simulink model "test_Dynamics_coupled_full_temp"  (R2021b)
settings: Solver=VariableStepAuto  StartTime=0.0  StopTime=10.0  RelTol=1e-3
InitFcn:
  | % ************** Initiate forces
  | % f0=[0;0;0;0;0;0];
  | % f0=[0;0;0;0;0;0;0];
  | f_0=[0;0;0];
  | f_m=[0;0];
  | f_e=[0;0;0;0;0;0];
  | % ************** Initiate states
  | q_m=[0;0];
  | q_dot_m=[0;0];
  | P=[0;0;0];
  | V_I0=[0;0;0];
  | % ************** Load main
  | %run(Main.m)
values from neighbouring files (symbols this model uses):
  diag_M = diagonalize(M_frak0, M_frak)    [Create_Robot.m]    (also in Main.m; diagonalize.m = zeros(6*(n+1),6*(n+1)); test_C_Main.m)
  iota0 = [1 0 0; 0 1 0;zeros(3,3);0 0 1]    [Create_Robot.m]    (also in Main.m = eye(6,6); test_C_Main.m)
  Xi_m_matrix = zeros(6*n,n)    [Create_Robot.m]    (also in Main.m; test_C_Main.m)
undefined symbols (not defined in the file or in its folder): Xi_m
settings Model: Creator=Bmmog  LastModifiedBy=Bmmog
settings SolverCC: AllowMultiTaskInputOutput=on

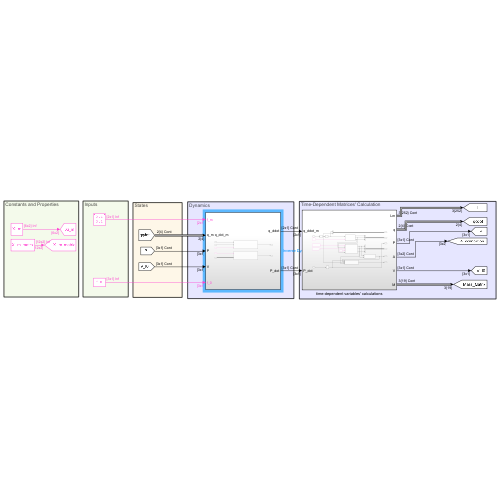
[thumbnail: Simulink's stored preview of the top-level diagram]
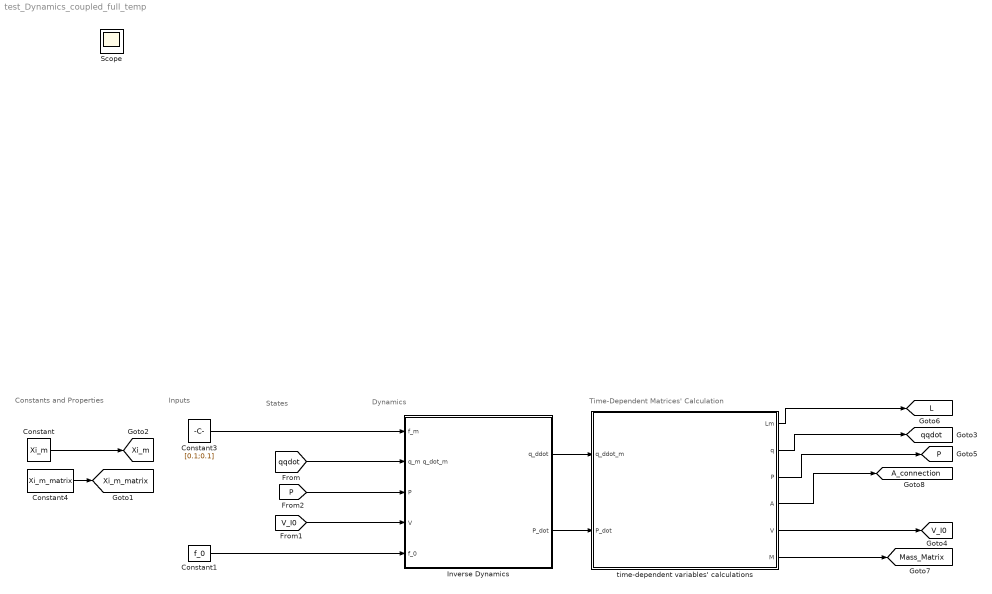
== system test_Dynamics_coupled_full_temp ==
  note: Time-Dependent Matrices' Calculation
  note: States
  note: Inputs
  note: Dynamics
  note: Constants and Properties
  Constant : Constant  Value=Xi_m  VectorParams1D=off
  Constant1 : Constant  Value=f_0  VectorParams1D=off
  Constant3 : Constant  Value=[0.1;0.1]  VectorParams1D=off
  Constant4 : Constant  Value=Xi_m_matrix  VectorParams1D=off
  Inverse Dynamics : Subsystem
  time-dependent variables' calculations : Subsystem
  Scope : Scope
  tag scope: A_connection=global, L=global, Mass_Matrix=global, P=global, V_I0=global, Xi_m=global, Xi_m_matrix=global, qqdot=global
  wires:
  Constant/1 -> [Xi_m]
  Constant4/1 -> [Xi_m_matrix]
  Constant3/1 -> Inverse Dynamics/1(f_m)
  time-dependent variables' calculations/6(M) -> [Mass_Matrix]
  time-dependent variables' calculations/1(Lm) -> [L]
  Inverse Dynamics/1(q_ddot) -> time-dependent variables' calculations/1(q_ddot_m)
  time-dependent variables' calculations/2(q) -> [qqdot]
  [qqdot] -> Inverse Dynamics/2(q_m q_dot_m)
  [V_I0] -> Inverse Dynamics/4(V)
  [P] -> Inverse Dynamics/3(P)
  time-dependent variables' calculations/3(P) -> [P]
  Constant1/1 -> Inverse Dynamics/5(f_0)
  time-dependent variables' calculations/4(A) -> [A_connection]
  time-dependent variables' calculations/5(V) -> [V_I0]
  Inverse Dynamics/2(P_dot) -> time-dependent variables' calculations/2(P_dot)

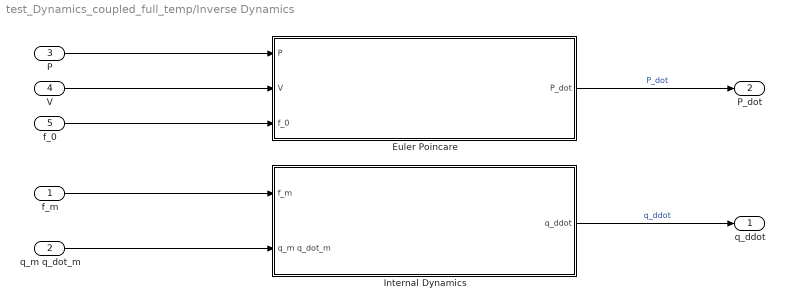
== system test_Dynamics_coupled_full_temp/Inverse Dynamics ==
  f_m : Inport
  q_m q_dot_m : Inport  Port=2
  P : Inport  Port=3
  V : Inport  Port=4
  f_0 : Inport  Port=5
  Euler Poincare : Subsystem
  Internal Dynamics : Subsystem
  q_ddot : Outport
  P_dot : Outport  Port=2
  wires:
  f_m/1 -> Internal Dynamics/1(f_m)
  Internal Dynamics/1(q_ddot) -> q_ddot/1  "q_ddot"
  q_m q_dot_m/1 -> Internal Dynamics/2(q_m q_dot_m)
  f_0/1 -> Euler Poincare/3(f_0)
  Euler Poincare/1(P_dot) -> P_dot/1  "P_dot"
  V/1 -> Euler Poincare/2(V)
  P/1 -> Euler Poincare/1(P)

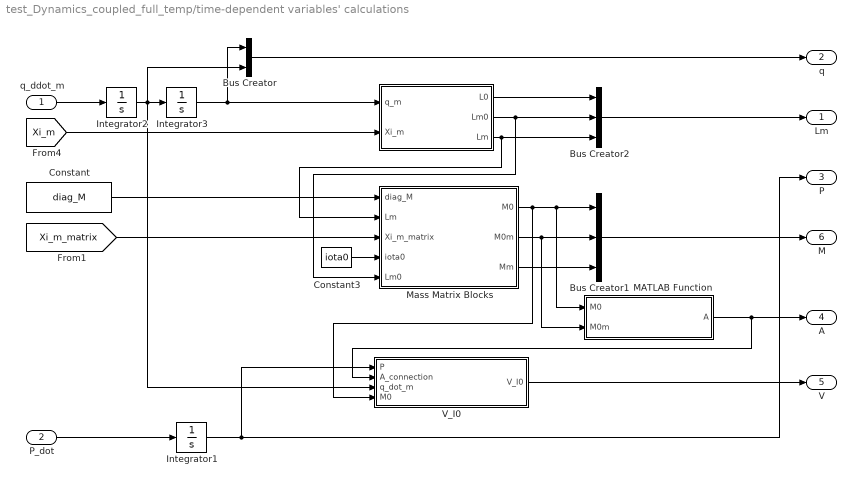
== system test_Dynamics_coupled_full_temp/time-dependent variables' calculations ==
  q_ddot_m : Inport
  P_dot : Inport  Port=2
  " " : MATLAB Function  TreatAsAtomicUnit=on
  Bus Creator : BusCreator  Inputs=2
  Bus Creator1 : BusCreator  Inputs=3
  Bus Creator2 : BusCreator  Inputs=3
  Constant : Constant  Value=diag_M  VectorParams1D=off
  Constant3 : Constant  Value=iota0  VectorParams1D=off
  Integrator1 : Integrator
  Integrator2 : Integrator
  Integrator3 : Integrator
  MATLAB Function : MATLAB Function  TreatAsAtomicUnit=on
  Mass Matrix Blocks : Subsystem
  V_I0 : MATLAB Function  TreatAsAtomicUnit=on
  Lm : Outport
  q : Outport  Port=2
  P : Outport  Port=3
  A : Outport  Port=4
  V : Outport  Port=5
  M : Outport  Port=6
  wires:
  Integrator2/1 -> V_I0/3(q_dot_m), Bus Creator/2, Integrator3/1
  q_ddot_m/1 -> Integrator2/1
  " "/1(L0) -> Bus Creator2/1
  " "/3(Lm) -> Mass Matrix Blocks/2(Lm), Bus Creator2/3
  " "/2(Lm0) -> Mass Matrix Blocks/5(Lm0), Bus Creator2/2
  Constant/1 -> Mass Matrix Blocks/1(diag_M)
  [Xi_m_matrix] -> Mass Matrix Blocks/3(Xi_m_matrix)
  [Xi_m] -> " "/2(Xi_m)
  Integrator3/1 -> Bus Creator/1, " "/1(q_m)
  Bus Creator/1 -> q/1
  Mass Matrix Blocks/1(M0) -> V_I0/4(M0), MATLAB Function/1(M0), Bus Creator1/1
  Mass Matrix Blocks/3(Mm) -> Bus Creator1/3
  Bus Creator1/1 -> M/1
  Mass Matrix Blocks/2(M0m) -> MATLAB Function/2(M0m), Bus Creator1/2
  MATLAB Function/1(A) -> V_I0/2(A_connection), A/1
  Constant3/1 -> Mass Matrix Blocks/4(iota0)
  Bus Creator2/1 -> Lm/1
  Integrator1/1 -> V_I0/1(P), P/1
  P_dot/1 -> Integrator1/1
  V_I0/1(V_I0) -> V/1

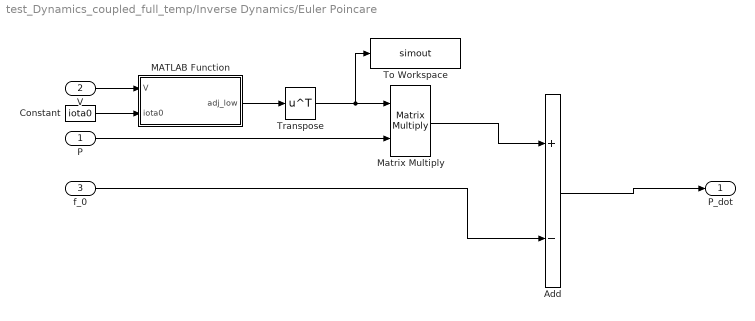
== system test_Dynamics_coupled_full_temp/Inverse Dynamics/Euler Poincare ==
  P : Inport
  V : Inport  Port=2
  f_0 : Inport  Port=3
  Add : Sum  Inputs=+-
  Constant : Constant  Value=iota0
  MATLAB Function : MATLAB Function  TreatAsAtomicUnit=on
  Matrix Multiply : Product  Multiplication=Matrix(*)
  To Workspace : ToWorkspace  VariableName=simout  SaveFormat=Timeseries  SampleTime=-1
  Transpose : Math  Operator=transpose  SaturateOnIntegerOverflow=on
  P_dot : Outport
  wires:
  P/1 -> Matrix Multiply/2
  MATLAB Function/1(adj_low) -> Transpose/1
  V/1 -> MATLAB Function/1(V)
  Transpose/1 -> To Workspace/1, Matrix Multiply/1
  Matrix Multiply/1 -> Add/1
  f_0/1 -> Add/2
  Add/1 -> P_dot/1
  Constant/1 -> MATLAB Function/2(iota0)

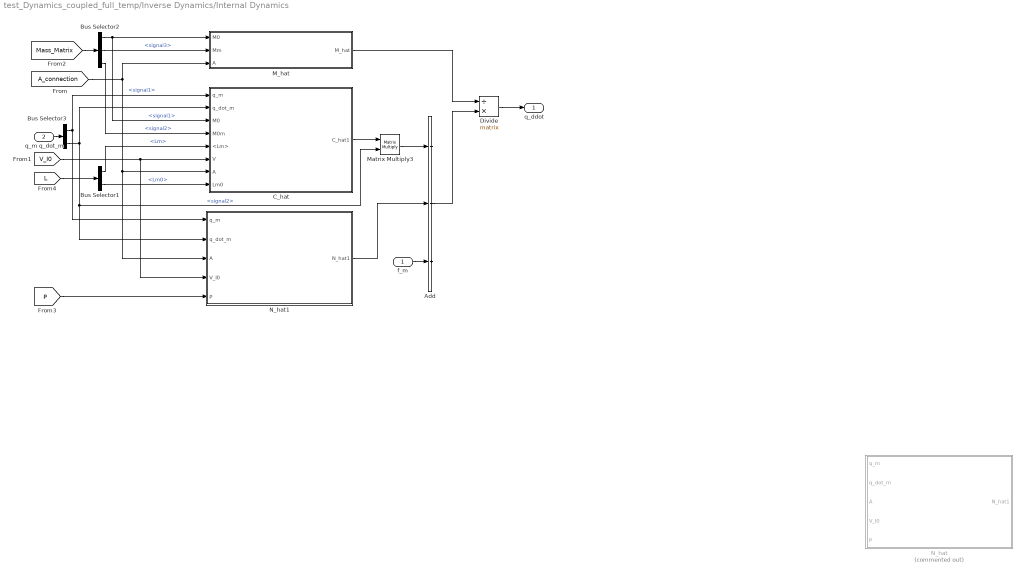
== system test_Dynamics_coupled_full_temp/Inverse Dynamics/Internal Dynamics ==
  f_m : Inport
  q_m q_dot_m : Inport  Port=2
  Add : Sum  Inputs=--+
  Bus Selector1 : BusSelector  OutputSignals=Lm,Lm0
  Bus Selector2 : BusSelector  OutputSignals=signal1,signal3,signal2
  Bus Selector3 : BusSelector  OutputSignals=signal1,signal2
  C_hat : Subsystem
  Divide : Product  Inputs=/*  Multiplication=Matrix(*)
  M_hat : MATLAB Function  TreatAsAtomicUnit=on
  Matrix Multiply3 : Product  Multiplication=Matrix(*)
  N_hat : Subsystem  Commented=on
  N_hat1 : Subsystem
  q_ddot : Outport
  wires:
  f_m/1 -> Add/3
  Divide/1 -> q_ddot/1
  q_m q_dot_m/1 -> Bus Selector3/1
  [Mass_Matrix] -> Bus Selector2/1
  [L] -> Bus Selector1/1
  C_hat/1(C_hat1) -> Matrix Multiply3/1
  Matrix Multiply3/1 -> Add/1
  Add/1 -> Divide/2
  Bus Selector3/2 -> C_hat/2(q_dot_m), N_hat1/2(q_dot_m), Matrix Multiply3/2  "<signal2>"
  Bus Selector3/1 -> C_hat/1(q_m), N_hat1/1(q_m)  "<signal1>"
  Bus Selector1/1 -> C_hat/5(<Lm>)  "<Lm>"
  M_hat/1(M_hat) -> Divide/1
  Bus Selector2/1 -> M_hat/1(M0), C_hat/3(M0)  "<signal1>"
  Bus Selector2/2 -> M_hat/2(Mm)  "<signal3>"
  [A_connection] -> N_hat1/3(A), C_hat/7(A), M_hat/3(A)
  Bus Selector2/3 -> C_hat/4(M0m)  "<signal2>"
  [V_I0] -> C_hat/6(V), N_hat1/4(V_I0)
  Bus Selector1/2 -> C_hat/8(Lm0)  "<Lm0>"
  [P] -> N_hat1/5(P)
  N_hat1/1(N_hat1) -> Add/2

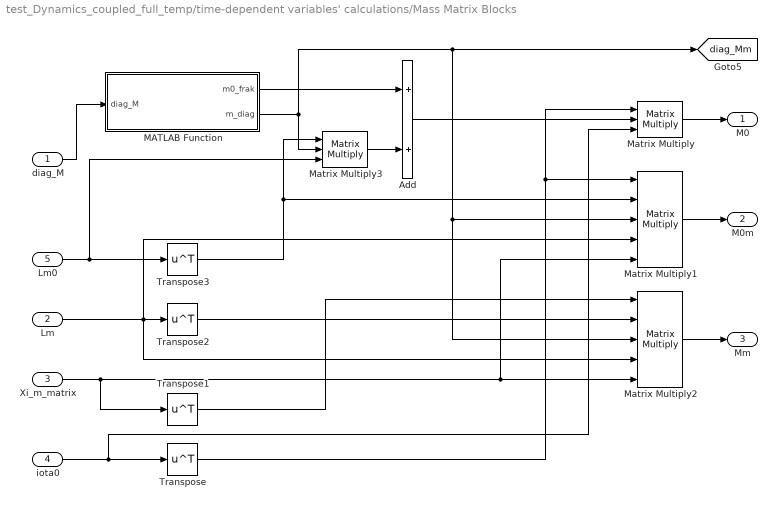
== system test_Dynamics_coupled_full_temp/time-dependent variables' calculations/Mass Matrix Blocks ==
  diag_M : Inport
  Lm : Inport  Port=2
  Xi_m_matrix : Inport  Port=3
  iota0 : Inport  Port=4
  Lm0 : Inport  Port=5
  Add : Sum
  MATLAB Function : MATLAB Function  TreatAsAtomicUnit=on
  Matrix Multiply : Product  Inputs=3  Multiplication=Matrix(*)
  Matrix Multiply1 : Product  Inputs=5  Multiplication=Matrix(*)
  Matrix Multiply2 : Product  Inputs=5  Multiplication=Matrix(*)
  Matrix Multiply3 : Product  Inputs=3  Multiplication=Matrix(*)
  Transpose{,1..3} (4 alike) : Math  Operator=transpose  SaturateOnIntegerOverflow=on
  M0 : Outport
  M0m : Outport  Port=2
  Mm : Outport  Port=3
  tag scope: diag_Mm=global
  wires:
  Matrix Multiply2/1 -> Mm/1
  Xi_m_matrix/1 -> Transpose1/1, Matrix Multiply1/5, Matrix Multiply2/5
  diag_M/1 -> MATLAB Function/1(diag_M)
  Lm/1 -> Matrix Multiply2/4, Matrix Multiply1/4, Transpose2/1
  Transpose1/1 -> Matrix Multiply2/1
  Transpose2/1 -> Matrix Multiply2/2
  MATLAB Function/2(m_diag) -> Matrix Multiply1/3, Matrix Multiply2/3, [diag_Mm], Matrix Multiply3/2
  Matrix Multiply1/1 -> M0m/1
  Matrix Multiply/1 -> M0/1
  iota0/1 -> Matrix Multiply/3, Transpose/1
  Transpose/1 -> Matrix Multiply/1, Matrix Multiply1/1
  Add/1 -> Matrix Multiply/2
  Matrix Multiply3/1 -> Add/2
  MATLAB Function/1(m0_frak) -> Add/1
  Lm0/1 -> Matrix Multiply3/3, Transpose3/1
  Transpose3/1 -> Matrix Multiply1/2, Matrix Multiply3/1

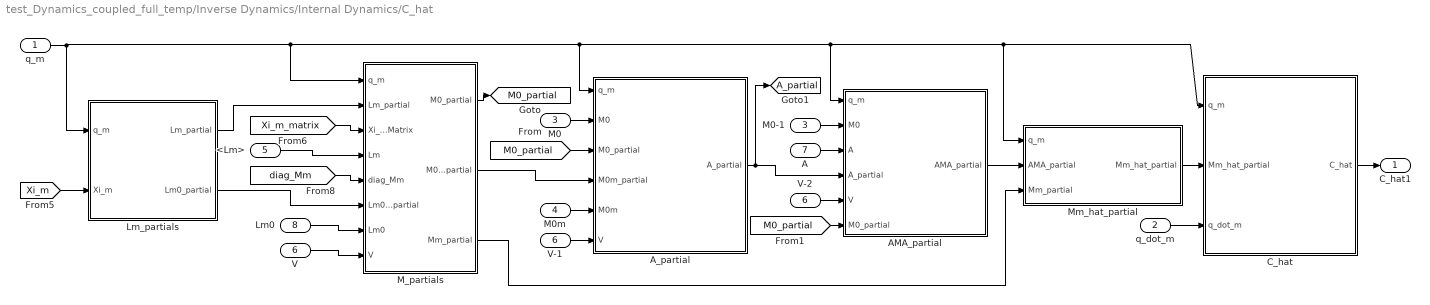
== system test_Dynamics_coupled_full_temp/Inverse Dynamics/Internal Dynamics/C_hat ==
  q_m : Inport
  q_dot_m : Inport  Port=2
  M0 : Inport  Port=3
  M0m : Inport  Port=4
  <Lm> : Inport  Port=5
  V : Inport  Port=6
  A : Inport  Port=7
  Lm0 : Inport  Port=8
  AMA_partial : MATLAB Function  TreatAsAtomicUnit=on
  A_partial : MATLAB Function  TreatAsAtomicUnit=on
  C_hat : MATLAB Function  TreatAsAtomicUnit=on
  Lm_partials : Subsystem
  M0-1 : InportShadow  Port=3
  M_partials : Subsystem
  Mm_hat_partial : MATLAB Function  TreatAsAtomicUnit=on
  V-1 : InportShadow  Port=6
  V-2 : InportShadow  Port=6
  C_hat1 : Outport
  tag scope: A_partial=global, M0_partial=global
  wires:
  C_hat/1(C_hat) -> C_hat1/1
  q_m/1 -> Mm_hat_partial/1(q_m), C_hat/1(q_m), AMA_partial/1(q_m), A_partial/1(q_m), M_partials/1(q_m), Lm_partials/1(q_m)
  q_dot_m/1 -> C_hat/3(q_dot_m)
  [Xi_m_matrix] -> M_partials/3(Xi_m_Matrix)
  <Lm>/1 -> M_partials/4(Lm)
  [diag_Mm] -> M_partials/5(diag_Mm)
  [Xi_m] -> Lm_partials/2(Xi_m)
  Lm_partials/1(Lm_partial) -> M_partials/2(Lm_partial)
  M_partials/3(Mm_partial) -> Mm_hat_partial/3(Mm_partial)
  Mm_hat_partial/1(Mm_hat_partial) -> C_hat/2(Mm_hat_partial)
  AMA_partial/1(AMA_partial) -> Mm_hat_partial/2(AMA_partial)
  A_partial/1(A_partial) -> [A_partial], AMA_partial/4(A_partial)
  M0/1 -> A_partial/2(M0)
  M0m/1 -> A_partial/5(M0m)
  V/1 -> M_partials/8(V)
  M_partials/2(M0m_partial) -> A_partial/4(M0m_partial)
  A/1 -> AMA_partial/3(A)
  Lm_partials/2(Lm0_partial) -> M_partials/6(Lm0_partial)
  Lm0/1 -> M_partials/7(Lm0)
  V-1/1 -> A_partial/6(V)
  V-2/1 -> AMA_partial/5(V)
  M0-1/1 -> AMA_partial/2(M0)
  M_partials/1(M0_partial) -> [M0_partial]
  [M0_partial] -> A_partial/3(M0_partial)
  [M0_partial] -> AMA_partial/6(M0_partial)

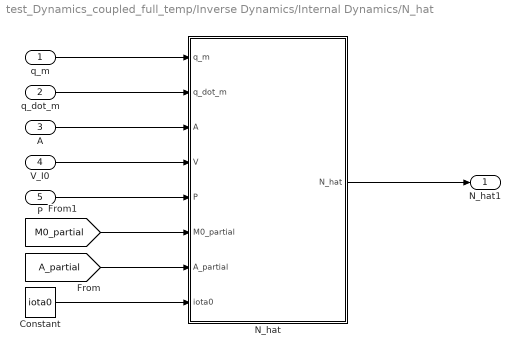
== system test_Dynamics_coupled_full_temp/Inverse Dynamics/Internal Dynamics/N_hat ==
  q_m : Inport
  q_dot_m : Inport  Port=2
  A : Inport  Port=3
  V_I0 : Inport  Port=4
  P : Inport  Port=5
  Constant : Constant  Value=iota0
  N_hat : MATLAB Function  TreatAsAtomicUnit=on
  N_hat1 : Outport
  wires:
  P/1 -> N_hat/5(P)
  [M0_partial] -> N_hat/6(M0_partial)
  N_hat/1(N_hat) -> N_hat1/1
  q_m/1 -> N_hat/1(q_m)
  q_dot_m/1 -> N_hat/2(q_dot_m)
  V_I0/1 -> N_hat/4(V)
  A/1 -> N_hat/3(A)
  [A_partial] -> N_hat/7(A_partial)
  Constant/1 -> N_hat/8(iota0)

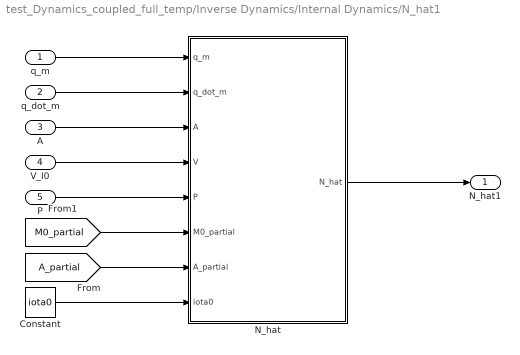
== system test_Dynamics_coupled_full_temp/Inverse Dynamics/Internal Dynamics/N_hat1 ==
  q_m : Inport
  q_dot_m : Inport  Port=2
  A : Inport  Port=3
  V_I0 : Inport  Port=4
  P : Inport  Port=5
  Constant : Constant  Value=iota0
  N_hat : MATLAB Function  TreatAsAtomicUnit=on
  N_hat1 : Outport
  wires:
  P/1 -> N_hat/5(P)
  [M0_partial] -> N_hat/6(M0_partial)
  N_hat/1(N_hat) -> N_hat1/1
  q_m/1 -> N_hat/1(q_m)
  q_dot_m/1 -> N_hat/2(q_dot_m)
  V_I0/1 -> N_hat/4(V)
  A/1 -> N_hat/3(A)
  [A_partial] -> N_hat/7(A_partial)
  Constant/1 -> N_hat/8(iota0)

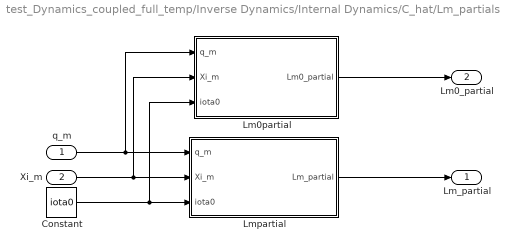
== system test_Dynamics_coupled_full_temp/Inverse Dynamics/Internal Dynamics/C_hat/Lm_partials ==
  q_m : Inport
  Xi_m : Inport  Port=2
  Constant : Constant  Value=iota0
  Lm0partial : MATLAB Function  TreatAsAtomicUnit=on
  Lmpartial : MATLAB Function  TreatAsAtomicUnit=on
  Lm_partial : Outport
  Lm0_partial : Outport  Port=2
  wires:
  Xi_m/1 -> Lm0partial/2(Xi_m), Lmpartial/2(Xi_m)
  q_m/1 -> Lm0partial/1(q_m), Lmpartial/1(q_m)
  Lmpartial/1(Lm_partial) -> Lm_partial/1
  Constant/1 -> Lm0partial/3(iota0), Lmpartial/3(iota0)
  Lm0partial/1(Lm0_partial) -> Lm0_partial/1

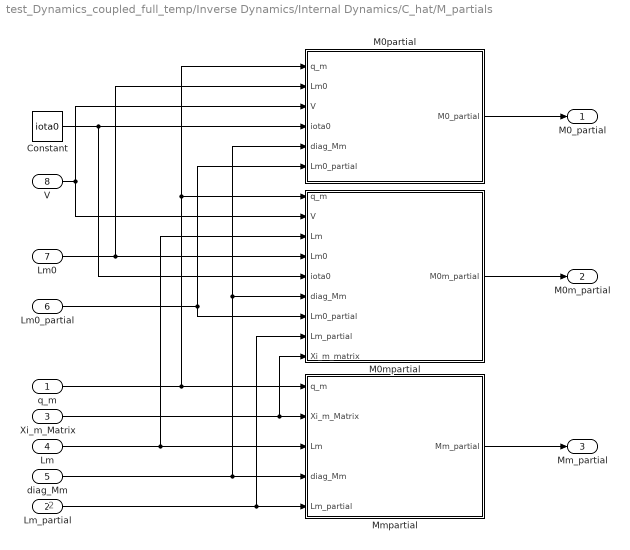
== system test_Dynamics_coupled_full_temp/Inverse Dynamics/Internal Dynamics/C_hat/M_partials ==
  note: 2
  q_m : Inport
  Lm_partial : Inport  Port=2
  Xi_m_Matrix : Inport  Port=3
  Lm : Inport  Port=4
  diag_Mm : Inport  Port=5
  Lm0_partial : Inport  Port=6
  Lm0 : Inport  Port=7
  V : Inport  Port=8
  " M0partial" : MATLAB Function  TreatAsAtomicUnit=on
  Constant : Constant  Value=iota0
  M0mpartial : MATLAB Function  TreatAsAtomicUnit=on
  Mmpartial : MATLAB Function  TreatAsAtomicUnit=on
  M0_partial : Outport
  M0m_partial : Outport  Port=2
  Mm_partial : Outport  Port=3
  wires:
  Xi_m_Matrix/1 -> M0mpartial/9(Xi_m_matrix), Mmpartial/2(Xi_m_Matrix)
  Lm/1 -> M0mpartial/3(Lm), Mmpartial/3(Lm)
  Mmpartial/1(Mm_partial) -> Mm_partial/1
  diag_Mm/1 -> " M0partial"/5(diag_Mm), M0mpartial/6(diag_Mm), Mmpartial/4(diag_Mm)
  M0mpartial/1(M0m_partial) -> M0m_partial/1
  Lm_partial/1 -> M0mpartial/8(Lm_partial), Mmpartial/5(Lm_partial)
  q_m/1 -> " M0partial"/1(q_m), M0mpartial/1(q_m), Mmpartial/1(q_m)
  " M0partial"/1(M0_partial) -> M0_partial/1
  Constant/1 -> " M0partial"/4(iota0), M0mpartial/5(iota0)
  Lm0_partial/1 -> " M0partial"/6(Lm0_partial), M0mpartial/7(Lm0_partial)
  Lm0/1 -> " M0partial"/2(Lm0), M0mpartial/4(Lm0)
  V/1 -> M0mpartial/2(V), " M0partial"/3(V)

== matlab function test_Dynamics_coupled_full_temp/time-dependent variables' calculations/MATLAB Function ==
  data: M0 input; M0m input; A output
function A=A_connection(M0,M0m)
% Compute the connection A from mass properties

A=M0\M0m;

== matlab function test_Dynamics_coupled_full_temp/Inverse Dynamics/Internal Dynamics/C_hat/Lm_partials/Lmpartial ==
  data: q_m input; Lm_partial output; Xi_m input; iota0 input
function Lm_partial  = Lm_partial(q_m,Xi_m,iota0)
% Calculates the C_hat_m matrix from base pose and arm joint angles

n=length(q_m);

% Find partial of Lm0 to joint angles
Lm_partial=zeros(6*n,6*n,n); % 6nx6xn
for i=1:n
    for j=1:n
        for k=1:n
            if j==k
                Lm_partial(6*(j-1)+1:6*(j-1)+6,6*(k-1)+1:6*(k-1)+6,i)=eye(6,6);
            elseif j>i && i>=k
                Lm_partial(6*(j-1)+1:6*j,6*(k-1)+1:6*k,i)=-Ad_frak(j,i+1,Xi_m,q_m)*adjoint_low(Xi_m(:,i),iota0)*Ad_frak(i,k,Xi_m,q_m); % equation 81 of TRO paper
            elseif i==j && i>=k
                Lm_partial(6*(j-1)+1:6*j,6*(k-1)+1:6*k,i)=-adjoint_low(Xi_m(:,i),iota0)*Ad_frak(i,k,Xi_m,q_m); % equation 81 of TRO paper
            else
                Lm_partial(6*(j-1)+1:6*(j-1)+6,6*(k-1)+1:6*(k-1)+6,i)=zeros(6,6);
            end

        end
    end
end

== matlab function test_Dynamics_coupled_full_temp/Inverse Dynamics/Internal Dynamics/C_hat/M_partials/ M0partial ==
  data: q_m input; M0_partial output; Lm0 input; V input; iota0 input; diag_Mm input; Lm0_partial input
function M0_partial = M0_partial(q_m,Lm0,V,iota0,diag_Mm,Lm0_partial)
% Calculates the C_hat_m matrix from base pose and arm joint angles

n=length(q_m);
b=length(V);

% Find partial of M0 to joint angles
M0_partial=zeros(b,b,n); %initiate
for i=1:n
    M0_partial(1:b,1:b,i)= iota0'*(transpose(Lm0_partial(1:end,1:end,i))*diag_Mm*Lm0+transpose(Lm0)*diag_Mm*Lm0_partial(1:end,1:end,i))*iota0; %6x6 %equation 117 of TRO
end

== matlab function test_Dynamics_coupled_full_temp/Inverse Dynamics/Internal Dynamics/C_hat/M_partials/M0mpartial ==
  data: q_m input; M0m_partial output; V input; Lm input; Lm0 input; iota0 input; diag_Mm input; Lm0_partial input; Lm_partial input; Xi_m_matrix input
function M0m_partial = M0m_partial(q_m,V,Lm,Lm0,iota0,diag_Mm,Lm0_partial,Lm_partial, Xi_m_matrix)
% Calculates the C_hat_m matrix from base pose and arm joint angles

n=length(q_m);
b=length(V);

% Find partial of M0m to joint angles
M0m_partial=zeros(b,n,n);
for i=1:n
    M0m_partial(1:b,1:n,i)= iota0'*((transpose(Lm0_partial(1:end,1:end,i))*diag_Mm*Lm+transpose(Lm0)*diag_Mm*Lm_partial(1:end,1:end,i)))*Xi_m_matrix; % equation 118 of TRO paper
end

== matlab function test_Dynamics_coupled_full_temp/time-dependent variables' calculations/Mass Matrix Blocks/MATLAB Function ==
  data: diag_M input; m0_frak output; m_diag output
function [m0_frak,m_diag]=m_frak_decomp(diag_M)
% Compute the Mass Matrix of the multibody system.
%   Output:
%   M0      Spacecraft mass matrix 
%   M0m
%   Mm      Manipulator mass matrix

%n=length(q_m);

m0_frak=diag_M(1:6,1:6);
m_diag=diag_M(7:end,7:end);

== matlab function test_Dynamics_coupled_full_temp/Inverse Dynamics/Internal Dynamics/C_hat/A_partial ==
  data: q_m input; A_partial output; M0 input; M0_partial input; M0m_partial input; M0m input; V input
function A_partial = A_partial(q_m,M0,M0_partial,M0m_partial,M0m,V)
% Calculates the C_hat_m matrix from base pose and arm joint angles

n=length(q_m);
b=length(V);

% Find partial of connection A to each joint angle
A_partial=zeros(b,n,n);

temp1=zeros(b,n);
temp2=zeros(b,n);
temp3=zeros(b,n);

for i=1:n
    temp1=M0\M0_partial(1:b,1:b,i);
    temp2=M0\M0m;
    temp3=M0\M0m_partial(1:b,1:n,i);
    A_partial(1:b,1:n,i)=temp1*temp2+temp3; % Equation 122
end

== matlab function test_Dynamics_coupled_full_temp/Inverse Dynamics/Internal Dynamics/C_hat/M_partials/Mmpartial ==
  data: q_m input; Mm_partial output; Xi_m_Matrix input; Lm input; diag_Mm input; Lm_partial input
function Mm_partial = Mm_partial(q_m,Xi_m_Matrix,Lm,diag_Mm,Lm_partial)
% Calculates the C_hat_m matrix from base pose and arm joint angles

n=length(q_m);

% find the non-generalized arm mass matrix'x derivative to joint angles
Mm_partial=zeros(n,n,n);
for i=1:n
    Mm_partial(1:n,1:n,i)=transpose(Xi_m_Matrix)*(transpose(Lm_partial(1:6*n,1:6*n,i))*diag_Mm*Lm + ...
        transpose(Lm)*diag_Mm*Lm_partial(1:6*n,1:6*n,i))*Xi_m_Matrix; %calcualte the derivative of not-augmented arm mass matrix from equation 120 of TRO paper
end

== matlab function test_Dynamics_coupled_full_temp/Inverse Dynamics/Internal Dynamics/C_hat/AMA_partial ==
  data: q_m input; AMA_partial output; M0 input; A input; A_partial input; V input; M0_partial input
function AMA_partial = AMA_partial(q_m,M0,A,A_partial,V,M0_partial)
% Calculates the C_hat_m matrix from base pose and arm joint angles

n=length(q_m);
b=length(V);

% find the temp intermediate term
AMA_partial=zeros(n,n,n);
for i=1:n
    AMA_partial(1:n,1:n,i)=transpose(A_partial(1:b,1:n,i))*M0*A+transpose(A)*M0_partial(1:b,1:b,i)*A+transpose(A)*M0*A_partial(1:b,1:n,i); %calcualte the derivative of not-augmented arm mass matrix from equation 121 of TRO paper
end

== matlab function test_Dynamics_coupled_full_temp/Inverse Dynamics/Internal Dynamics/C_hat/Mm_hat_partial ==
  data: q_m input; AMA_partial input; Mm_hat_partial output; Mm_partial input
function Mm_hat_partial = Mm_hat_partial(q_m, AMA_partial, Mm_partial)
% Calculates the C_hat_m matrix from base pose and arm joint angles

n=length(q_m);

% find the generalized arm mass matrix'x derivative to joint angles
Mm_hat_partial=zeros(n,n,n);
for i=1:n
    Mm_hat_partial(1:n,1:n,i)=Mm_partial(1:n,1:n,i)-AMA_partial(1:n,1:n,i); %calcualte the derivative of augmented arm mass matrix from equation 119 of TRO paper
end

== matlab function test_Dynamics_coupled_full_temp/time-dependent variables' calculations/V_I0 ==
  data: P input; A_connection input; q_dot_m input; M0 input; V_I0 output
function V_I0=V_I0(P,A_connection,q_dot_m,M0)
% Find the spaccecraft velocity V_I0
% M0_inv=inv(M0);
% temp=P-transpose(A_connection)*q_dot_m;
V_I0=M0\P-A_connection*q_dot_m;

== matlab function test_Dynamics_coupled_full_temp/Inverse Dynamics/Internal Dynamics/N_hat1/N_hat ==
  data: N_hat output; q_m input; q_dot_m input; A input; V input; P input; M0_partial input; A_partial input; iota0 input
function N_hat = N_hat(q_m,q_dot_m,A,V,P,M0_partial, A_partial, iota0)
% Calculates the N_hat_m matrix from base pose and arm joint angles

n=length(q_m);
b=length(V);

%Form N_hat from equation 19 of ACC paper
N_temp1=zeros(n,b); N_temp2=zeros(n,b); N_temp3=zeros(n,b);

for i=1:n
    N_temp1=N_temp1+transpose(squeeze(A_partial(1:b,1:n,i)).*q_dot_m(i)); % transpose of (bxn times 1x1)
    N_temp2(i,1:b)=transpose(q_dot_m)*transpose(squeeze(A_partial(1:b,1:n,i))); %1xn times nxb
    N_temp3(i,1:b)=0.5*transpose(P)*squeeze(M0_partial(1:b,1:b,i)); % 1xb times bxb
end

N_hat=transpose(A)*transpose(adjoint_low(V,iota0))*P-N_temp1*P+N_temp2*P+N_temp3*P;

== matlab function test_Dynamics_coupled_full_temp/Inverse Dynamics/Euler Poincare/MATLAB Function ==
  data: V input; adj_low output; iota0 input
function adj_low = adj_low(V, iota0)
% calculates the adjoint corresponding to the Lie bracket of vector V and ()
adj_low = adjoint_low(V,iota0);

== matlab function test_Dynamics_coupled_full_temp/Inverse Dynamics/Internal Dynamics/C_hat/C_hat ==
  data: q_m input; Mm_hat_partial input; q_dot_m input; C_hat output
function C_hat = C_hat(q_m, Mm_hat_partial,q_dot_m)
% Calculates the C_hat_m matrix from base pose and arm joint angles

n=length(q_m);


% Calculate C_hat matrix
C_temp1=zeros(n,n);
C_temp2=zeros(n,n);
C_hat=zeros(n,n);
for i=1:n
    C_temp1=C_temp1+Mm_hat_partial(1:n,1:n,i).*q_dot_m(i); % nxn by scalar
    C_temp2(i,1:n)=0.5*transpose(q_dot_m)*Mm_hat_partial(1:n,1:n,i); %1xn by nxn 
end

C_hat=C_temp1-C_temp2;

== matlab function test_Dynamics_coupled_full_temp/Inverse Dynamics/Internal Dynamics/C_hat/Lm_partials/Lm0partial ==
  data: q_m input; Lm0_partial output; Xi_m input; iota0 input
function Lm0_partial = Lm0_partial(q_m,Xi_m,iota0)
% Calculates the C_hat_m matrix from base pose and arm joint angles

n=length(q_m);

% Find partial of Lm to joint angles
Lm0_partial=zeros(6*n,6,n); % 6nx6xn
for i=1:n
    for j=1:n
        Lm0_partial(6*(j-1)+1:6*j,1:6,i)=Ad_partial(j,1,i,Xi_m,q_m,iota0); % equation 114 of TRO paper
    end
end

== matlab function test_Dynamics_coupled_full_temp/Inverse Dynamics/Internal Dynamics/M_hat ==
  data: M0 input; Mm input; A input; M_hat output
function M_hat =M_hat(M0,Mm,A)
% Compute the Mass Matrix of the multibody system.
%   Input:
%   M0      Spacecraft mass matrix 
%   M0m     Coupling
%   Mm      Manipulator mass matrix

% Calculate M_hat
M_hat=Mm-transpose(A)*M0*A;


end

== matlab function test_Dynamics_coupled_full_temp/Inverse Dynamics/Internal Dynamics/N_hat/N_hat ==
  data: N_hat output; q_m input; q_dot_m input; A input; V input; P input; M0_partial input; A_partial input; iota0 input
function N_hat = N_hat(q_m,q_dot_m,A,V,P,M0_partial, A_partial, iota0)
% Calculates the N_hat_m matrix from base pose and arm joint angles

n=length(q_m);
b=length(V);

%Form N_hat from equation 19 of ACC paper
N_temp1=zeros(n,b); N_temp2=zeros(n,b); N_temp3=zeros(n,b);

for i=1:n
    N_temp1=N_temp1+transpose(squeeze(A_partial(1:b,1:n,i)).*q_dot_m(i)); % transpose of (bxn times 1x1)
    N_temp2(i,1:b)=transpose(q_dot_m)*transpose(squeeze(A_partial(1:b,1:n,i))); %1xn times nxb
    N_temp3(i,1:b)=0.5*transpose(P)*squeeze(M0_partial(1:b,1:b,i)); % 1xb times bxb
end

N_hat=transpose(A)*transpose(adjoint_low(V,iota0))*P-N_temp1*P+N_temp2*P+N_temp3*P;

== matlab function test_Dynamics_coupled_full_temp/time-dependent variables' calculations/  ==
  data: q_m input; L0 output; Lm0 output; Lm output; Xi_m input
function [L0,Lm0,Lm] =L_calculator(q_m,Xi_m)
% Calculates the time-dependent L matrix
n=length(q_m);
L=zeros(6*(n+1),6*(n+1));
% Compute M_frak for ith body
% Calculate L matrix
for i=1:n+1
    for j=1:n+1
        if i>j
            Ad_temp=eye(6);
            for k=j:i-1
                Ad_temp=Adjoint(g_Matrix(-Xi_m(:,k),q_m(k)))*Ad_temp;
            end
            L(6*(i-1)+1:6*(i-1)+6,6*(j-1)+1:6*(j-1)+6)=Ad_temp;
        elseif i==j
            L(6*(i-1)+1:6*(i-1)+6,6*(j-1)+1:6*(j-1)+6)=eye(6);
        elseif i<j
            L(6*(i-1)+1:6*(i-1)+6,6*(j-1)+1:6*(j-1)+6)=zeros(6);
        end
    end
end

L0=L(1:6,1:6);
Lm0=L(7:end,1:6);
Lm=L(7:end,7:end);

end
